simulink model "net"  (R2013a)
settings: Solver=ode45  StartTime=0.0  StopTime=inf  RelTol=1e-3
libraries: instrumentlib x2, simulink x1, utility x1
settings Model: Creator=x86  LastModifiedBy=x86
settings HardwareCC: ProdLargestAtomicInteger=Long  ProdLargestAtomicFloat=Double  ProdEndianess=LittleEndian  ProdHWDeviceType=ARM Compatible->ARM Cortex

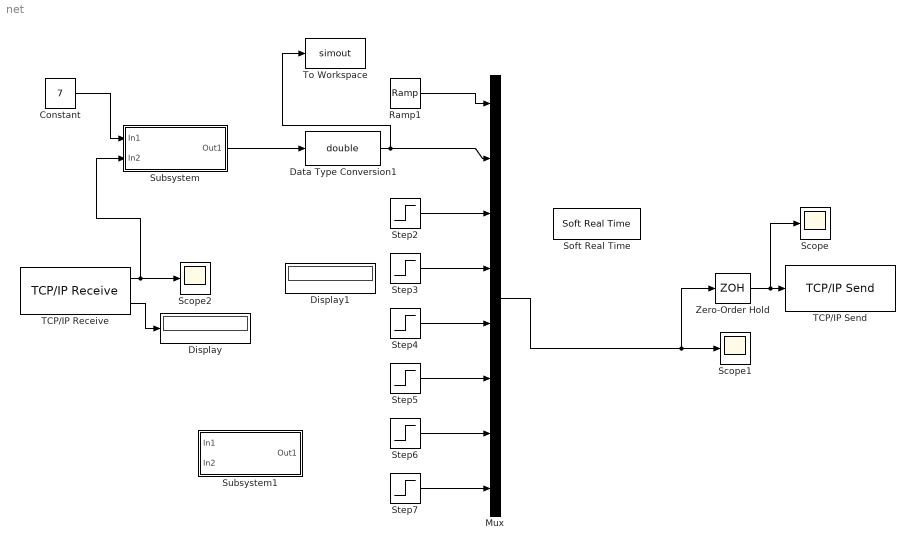
== system net ==
  Constant : Constant  Value=7  VectorParams1D=off  OutDataTypeStr=double
  Data Type Conversion1 : DataTypeConversion  OutDataTypeStr=double
  Display : Display
  Display1 : Display
  Mux : Mux  Inputs=8
  Ramp1 : simulink/Sources/Ramp  slope=1  start=0  X0=0
  Scope : Scope
      settings: TimeRange=0.002601626016259573  YMin=7.418012903225804  YMax=7.622812903225805
  Scope1 : Scope
      settings: TimeRange=10  YMin=0  YMax=400
  Scope2 : Scope
      settings: TimeRange=10  YMin=0  YMax=400  SaveName=ScopeData2
  Soft Real Time : utility/Soft Real Time  x=1
  Step2 : Step  After=3  SampleTime=0
  Step3 : Step  After=4  SampleTime=0
  Step4 : Step  After=5  SampleTime=0
  Step5 : Step  After=6  SampleTime=0
  Step6 : Step  After=7  SampleTime=0
  Step7 : Step  After=8  SampleTime=0
  Subsystem : Subsystem
  Subsystem1 : Subsystem
  TCP/IP Receive : instrumentlib/TCP//IP Receive  Host=192.168.7.2  Port=10000  DataSize="[1  1]"  EnableBlockingMode=off  Timeout=10  SampleTime=1  DataType=single  ByteOrder=LittleEndian
  TCP/IP Send : instrumentlib/TCP//IP Send  Host=192.168.7.2  Port=10000  EnableBlockingMode=off  Timeout=10000  ByteOrder=LittleEndian
  To Workspace : ToWorkspace  VariableName=simout  SampleTime=-1  SaveFormat=Timeseries
  Zero-Order Hold : ZeroOrderHold
  wires:
  Mux/1 -> Zero-Order Hold/1, Scope1/1
  TCP/IP Receive/2 -> Display/1
  Zero-Order Hold/1 -> Scope/1, TCP/IP Send/1
  Ramp1/1 -> Mux/1
  Step2/1 -> Mux/3
  Step3/1 -> Mux/4
  Step4/1 -> Mux/5
  Step5/1 -> Mux/6
  Step6/1 -> Mux/7
  Step7/1 -> Mux/8
  Data Type Conversion1/1 -> Mux/2, To Workspace/1
  Constant/1 -> Subsystem/1(In1)
  TCP/IP Receive/1 -> Scope2/1, Subsystem/2(In2)
  Subsystem/1(Out1) -> Data Type Conversion1/1

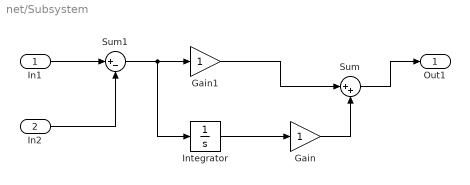
== system net/Subsystem ==
  In1 : Inport
  In2 : Inport  Port=2
  Gain : Gain
  Gain1 : Gain
  Integrator : Integrator
  Sum : Sum  Inputs=|++
  Sum1 : Sum  Inputs=|+-
  Out1 : Outport
  wires:
  Integrator/1 -> Gain/1
  Gain/1 -> Sum/2
  Gain1/1 -> Sum/1
  Sum/1 -> Out1/1
  Sum1/1 -> Integrator/1, Gain1/1
  In2/1 -> Sum1/2
  In1/1 -> Sum1/1

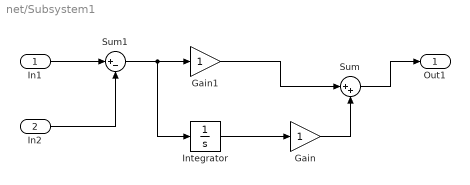
== system net/Subsystem1 ==
  In1 : Inport
  In2 : Inport  Port=2
  Gain : Gain
  Gain1 : Gain
  Integrator : Integrator
  Sum : Sum  Inputs=|++
  Sum1 : Sum  Inputs=|+-
  Out1 : Outport
  wires:
  Integrator/1 -> Gain/1
  Gain/1 -> Sum/2
  Gain1/1 -> Sum/1
  Sum/1 -> Out1/1
  Sum1/1 -> Integrator/1, Gain1/1
  In2/1 -> Sum1/2
  In1/1 -> Sum1/1
